simulink model "Lab2partA"  (R2013b)
settings: Solver=ode45  StartTime=0.0  StopTime=12.8  RelTol=1e-3
settings Model: Creator=BenjaminMoshirian  LastModifiedBy=Christina
settings DataIOCC: SignalLoggingSaveFormat=ModelDataLogs
settings DebuggingCC: UnderspecifiedInitializationDetection=Simplified  MultiTaskDSMMsg=warning  MultiTaskCondExecSysMsg=none
settings RTWCC: IncludeERTFirstTime=on
settings GRTTargetCC: CodeReplacementLibrary=None  CPPClassGenCompliant=on

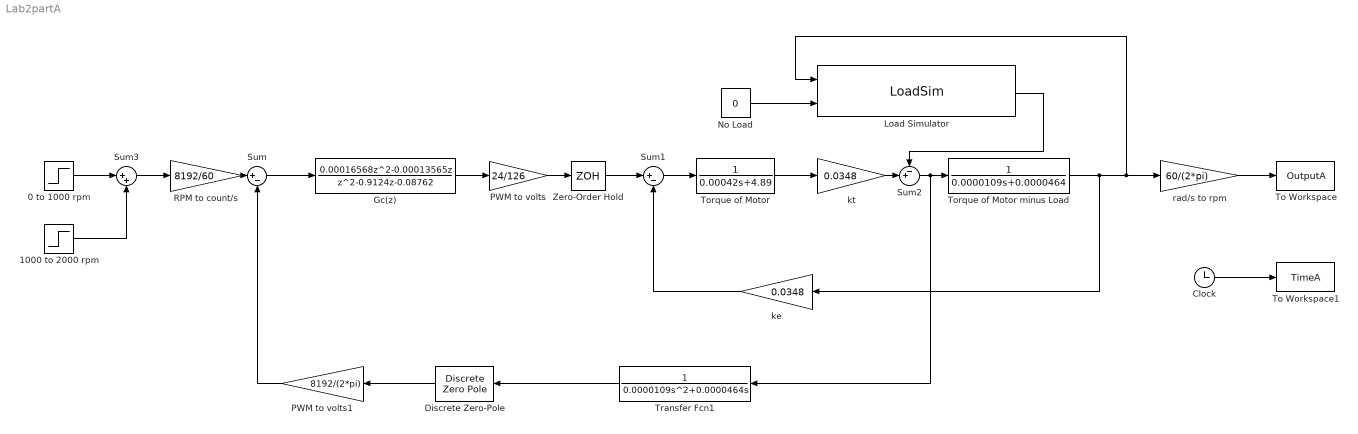
== system Lab2partA ==
  0 to 1000 rpm : Step  Time=0  After=1000  SampleTime=0.008
  1000 to 2000 rpm : Step  Time=3.456  After=1000  SampleTime=0.008
  Clock : Clock
  Discrete Zero-Pole : DiscreteZeroPole  Poles=[0]  Gain=1/0.008  SampleTime=0.008
  Gc(z) : DiscreteTransferFcn  Numerator=[0.00016568 -0.00013565 0]  Denominator=[1 -0.9124 -0.08762]  SampleTime=0.008
  Load Simulator : S-Function  InitFcn=try, set_param(gcb,'FunctionName','LoadSim'), end  FunctionName=LoadSim  SFunctionModules=LoadSim_wrapper  EnableBusSupport=off  mask(S-Function Builder){}
      mask help: Simulink:masks:SFunctionBuilder_MD
      mask init:
      | val = [[.9  0.75 0.75 1 1 .9 .9 1]',[1 1 0.75 0.75 .9 .9 1 .9]'];try , sys = get_param(gcb,'SfunBuilderFcnName');if isempty(sys), sys = get_param(gcb,'FunctionName'); end,catch, sys = get_param(gcb,'FunctionName'); end
      settings: CopyFcn=set_param(gcbh,'LinkStatus','none')  PreSaveFcn=try, set_param(gcb,'FunctionName','LoadSim'), end  OpenFcn=sfunctionwizard(gcbh)
      mask Display: plot(val(:,1),val(:,2)),disp(sys), port_label('input',1,'u0'), port_label('input',2,'u1'), port_label('output',1,'y0')
  No Load : Constant  Value=0
  PWM to volts : Gain  Gain=24/126
  PWM to volts1 : Gain  Gain=8192/(2*pi)
  RPM to count/s : Gain  Gain=8192/60
  Sum : Sum  Inputs=|+-
  Sum1 : Sum  Inputs=|+-
  Sum2 : Sum  Inputs=-+|
  Sum3 : Sum  Inputs=|++  SampleTime=0.008
  To Workspace : ToWorkspace  VariableName=OutputA  SampleTime=-1
  To Workspace1 : ToWorkspace  VariableName=TimeA  SampleTime=-1
  Torque of Motor : TransferFcn  Denominator=[0.00042 4.89]
  Torque of Motor minus Load : TransferFcn  Denominator=[0.0000109 0.0000464]
  Transfer Fcn1 : TransferFcn  Denominator=[0.0000109 0.0000464 0]
  Zero-Order Hold : ZeroOrderHold  SampleTime=0.008
  ke : Gain  Gain=0.0348
  kt : Gain  Gain=0.0348
  rad/s to rpm : Gain  Gain=60/(2*pi)
  wires:
  RPM to count/s/1 -> Sum/1
  Sum/1 -> Gc(z)/1
  Gc(z)/1 -> PWM to volts/1
  Zero-Order Hold/1 -> Sum1/1
  Sum1/1 -> Torque of Motor/1
  Torque of Motor/1 -> kt/1
  kt/1 -> Sum2/2
  Sum2/1 -> Transfer Fcn1/1, Torque of Motor minus Load/1
  ke/1 -> Sum1/2
  Torque of Motor minus Load/1 -> Load Simulator/1, rad/s to rpm/1, ke/1
  Load Simulator/1 -> Sum2/1
  Clock/1 -> To Workspace1/1
  PWM to volts/1 -> Zero-Order Hold/1
  Discrete Zero-Pole/1 -> PWM to volts1/1
  PWM to volts1/1 -> Sum/2
  rad/s to rpm/1 -> To Workspace/1
  Sum3/1 -> RPM to count/s/1
  No Load/1 -> Load Simulator/2
  0 to 1000 rpm/1 -> Sum3/1
  1000 to 2000 rpm/1 -> Sum3/2
  Transfer Fcn1/1 -> Discrete Zero-Pole/1
